simulink model "Simulation"  (R2025b)
settings: Solver=ode4  StartTime=0.0  StopTime=60  FixedStep=Ts  RelTol=1e-3
undefined symbols (not defined in the file or in its folder): A_SS_FD1, A_SS_FD3, A_zeta_f, A_zeta_tau, B_SS_FD1, B_SS_FD3, C_SS_FD1, C_SS_FD3, C_zeta_f, C_zeta_tau, D_SS_FD1, D_SS_FD3, eigs_NDO_force, eigs_NDO_torque, F1, F2, g_vec, inertia_factor, J, m, mass_factor, NDOB_force, NDOB_torque, period, radius, ReferenceTypeNumber, speed, Th_lower, Th_upper, Ts, Ts_hw, x0_FD1
libraries: simulink x9, dspstat3 x2
(part 1 of 2)
settings Model: SimulationMode=accelerator  SILPILSystemUnderTest=refmodels  Creator=baldo  LastModifiedBy=robyd
settings DebuggingCC: UnconnectedInputMsg=warning  UnconnectedOutputMsg=warning  UnconnectedLineMsg=warning
settings ModelReferenceCC: EnableRefExpFcnMdlSchedulingChecks=on
settings RTWCC: GPUComputeCapability=3.5  DLArmComputeVersion=19.05

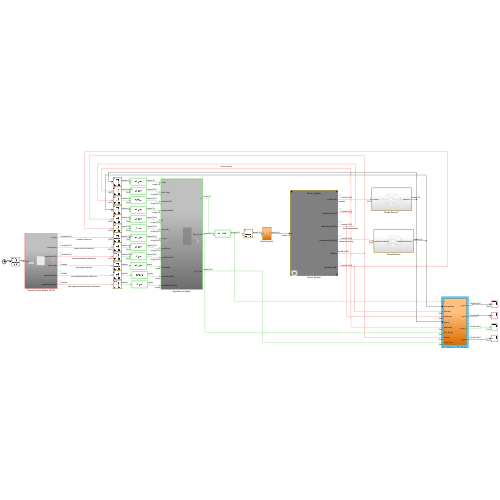
[thumbnail: Simulink's stored preview of the top-level diagram]
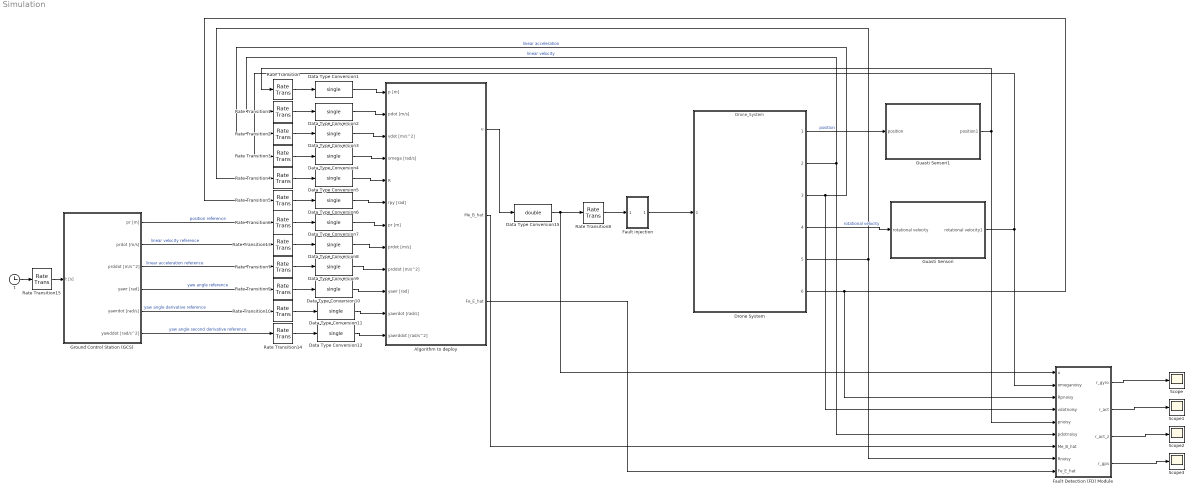
== system Simulation ==
  Algorithm to deploy : Subsystem
  Data Type Conversion{1..12} (12 alike) : DataTypeConversion  OutDataTypeStr=single  SaturateOnIntegerOverflow=off  RndMeth=Floor
  Data Type Conversion15 : DataTypeConversion  OutDataTypeStr=double  SaturateOnIntegerOverflow=off  RndMeth=Floor
  Drone System : ModelReference  ModelNameDialog=Drone_System  ModelReferenceVersion=9.10  CopyOfModelProtected=on
  Fault Detection (FD) Module : Subsystem
  Fault injection : Subsystem
  Ground Control Station (GCS) : Subsystem
  Guasti Sensori : Subsystem
  Guasti Sensori1 : Subsystem
  Rate Transition{,1..7,9..10,13..14} (12 alike) : RateTransition  OutPortSampleTime=Ts_hw
  Rate Transition15 : RateTransition  OutPortSampleTime=Ts
  Rate Transition8 : RateTransition  OutPortSampleTime=Ts
  Scope{,1..3} (4 alike) : Scope
      Scope settings: ActiveDisplayYMinimum=-1  ActiveDisplayYMaximum=1  DataLoggingVariableName=ScopeData5
      Scope1 settings: ActiveDisplayYMinimum=-1  ActiveDisplayYMaximum=1  DataLoggingVariableName=ScopeData7
      Scope2 settings: ActiveDisplayYMinimum=-1  ActiveDisplayYMaximum=1  DataLoggingVariableName=ScopeData8
      Scope3 settings: ActiveDisplayYMinimum=-1  ActiveDisplayYMaximum=1  DataLoggingVariableName=ScopeData9
  t : Clock
  wires:
  Algorithm to deploy/1(u) -> Data Type Conversion15/1
  Rate Transition/1 -> Data Type Conversion1/1
  Rate Transition1/1 -> Data Type Conversion2/1
  Rate Transition2/1 -> Data Type Conversion3/1
  Rate Transition3/1 -> Data Type Conversion4/1
  Rate Transition4/1 -> Data Type Conversion5/1
  Rate Transition5/1 -> Data Type Conversion6/1
  Rate Transition6/1 -> Data Type Conversion7/1
  Rate Transition13/1 -> Data Type Conversion8/1
  Rate Transition7/1 -> Data Type Conversion9/1
  Rate Transition9/1 -> Data Type Conversion10/1
  Rate Transition10/1 -> Data Type Conversion11/1
  Rate Transition14/1 -> Data Type Conversion12/1
  t/1 -> Rate Transition15/1
  Ground Control Station (GCS)/1(pr [m]) -> Rate Transition6/1  "position reference"
  Ground Control Station (GCS)/2(prdot [m/s]) -> Rate Transition13/1  "linear velocity reference"
  Ground Control Station (GCS)/3(prddot [m/s^2]) -> Rate Transition7/1  "linear acceleration reference"
  Ground Control Station (GCS)/4(yawr [rad]) -> Rate Transition9/1  "yaw angle reference"
  Ground Control Station (GCS)/5(yawrdot [rad/s]) -> Rate Transition10/1  "yaw angle derivative reference"
  Ground Control Station (GCS)/6(yawddot [rad/s^2]) -> Rate Transition14/1  "yaw angle second derivative reference"
  Data Type Conversion1/1 -> Algorithm to deploy/1(p [m])
  Data Type Conversion2/1 -> Algorithm to deploy/2(pdot [m/s])
  Data Type Conversion3/1 -> Algorithm to deploy/3(vdot [m/s^2])
  Data Type Conversion4/1 -> Algorithm to deploy/4(omega [rad/s])
  Data Type Conversion5/1 -> Algorithm to deploy/5(R)
  Data Type Conversion6/1 -> Algorithm to deploy/6(rpy [rad])
  Data Type Conversion7/1 -> Algorithm to deploy/7(pr [m])
  Data Type Conversion8/1 -> Algorithm to deploy/8(prdot [m/s])
  Data Type Conversion9/1 -> Algorithm to deploy/9(prddot [m/s^2])
  Data Type Conversion10/1 -> Algorithm to deploy/10(yawr [rad])
  Data Type Conversion11/1 -> Algorithm to deploy/11(yawrdot [rad/s])
  Data Type Conversion12/1 -> Algorithm to deploy/12(yawrddot [rad/s^2])
  Data Type Conversion15/1 -> Fault Detection (FD) Module/1(u), Rate Transition8/1
  Rate Transition15/1 -> Ground Control Station (GCS)/1(t [s])
  Drone System/2 -> Rate Transition1/1, Fault Detection (FD) Module/6(pdotnoisy)  "linear velocity"
  Drone System/3 -> Fault Detection (FD) Module/4(vdotnoisy), Rate Transition2/1  "linear acceleration"
  Drone System/5 -> Rate Transition4/1, Fault Detection (FD) Module/8(Rnoisy)
  Rate Transition8/1 -> Fault injection/1(In1)
  Fault injection/1(Out1) -> Drone System/1
  Drone System/4 -> Guasti Sensori/1(rotational velocity)  "rotational velocity"
  Guasti Sensori/1(rotational velocity1) -> Rate Transition3/1, Fault Detection (FD) Module/2(omeganoisy)
  Drone System/6 -> Fault Detection (FD) Module/3(Rpnoisy), Rate Transition5/1
  Drone System/1 -> Guasti Sensori1/1(position)  "position"
  Guasti Sensori1/1(position1) -> Fault Detection (FD) Module/5(pnoisy), Rate Transition/1
  Fault Detection (FD) Module/1(r_gyro) -> Scope/1
  Fault Detection (FD) Module/2(r_act) -> Scope1/1
  Fault Detection (FD) Module/3(r_act_z) -> Scope2/1
  Fault Detection (FD) Module/4(r_gps) -> Scope3/1
  Algorithm to deploy/2(Me_B_hat) -> Fault Detection (FD) Module/7(Me_B_hat)
  Algorithm to deploy/3(Fe_E_hat) -> Fault Detection (FD) Module/9(Fe_E_hat)

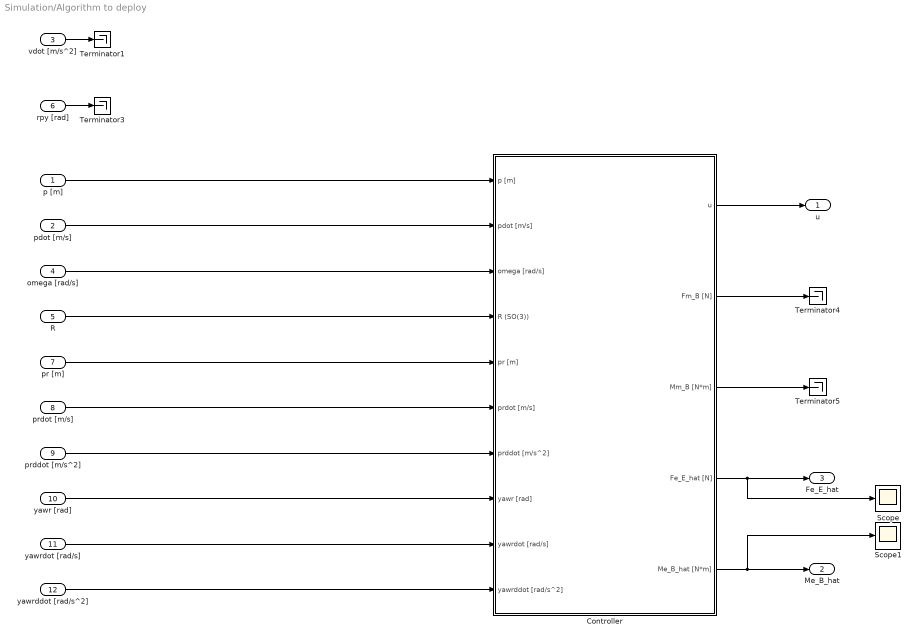
== system Simulation/Algorithm to deploy ==
  p [m] : Inport  OutDataTypeStr=single
  pdot [m/s] : Inport  Port=2  OutDataTypeStr=single
  vdot [m/s^2] : Inport  Port=3  OutDataTypeStr=single
  omega [rad/s] : Inport  Port=4  OutDataTypeStr=single
  R : Inport  Port=5  OutDataTypeStr=single
  rpy [rad] : Inport  Port=6  OutDataTypeStr=single
  pr [m] : Inport  Port=7  OutDataTypeStr=single
  prdot [m/s] : Inport  Port=8  OutDataTypeStr=single
  prddot [m/s^2] : Inport  Port=9  OutDataTypeStr=single
  yawr [rad] : Inport  Port=10  OutDataTypeStr=single
  yawrdot [rad/s] : Inport  Port=11  OutDataTypeStr=single
  yawrddot [rad/s^2] : Inport  Port=12  OutDataTypeStr=single
  Controller : Subsystem
  Scope : Scope
      settings: ActiveDisplayYMinimum=-18.049574136734009  ActiveDisplayYMaximum=25.171024560928345
  Scope1 : Scope
      settings: ActiveDisplayYMinimum=-0.31069509871304035  ActiveDisplayYMaximum=1.0718367416411638  DataLoggingVariableName=ScopeData2
  Terminator{1,3..5} (4 alike) : Terminator
  u : Outport  OutDataTypeStr=single
  Me_B_hat : Outport  Port=2  OutDataTypeStr=single
  Fe_E_hat : Outport  Port=3  OutDataTypeStr=single
  wires:
  vdot [m/s^2]/1 -> Terminator1/1
  rpy [rad]/1 -> Terminator3/1
  p [m]/1 -> Controller/1(p [m])
  pdot [m/s]/1 -> Controller/2(pdot [m/s])
  omega [rad/s]/1 -> Controller/3(omega [rad/s])
  R/1 -> Controller/4(R (SO(3)))
  pr [m]/1 -> Controller/5(pr [m])
  prdot [m/s]/1 -> Controller/6(prdot [m/s])
  prddot [m/s^2]/1 -> Controller/7(prddot [m/s^2])
  yawr [rad]/1 -> Controller/8(yawr [rad])
  yawrdot [rad/s]/1 -> Controller/9(yawrdot [rad/s])
  yawrddot [rad/s^2]/1 -> Controller/10(yawrddot [rad/s^2])
  Controller/1(u) -> u/1
  Controller/2(Fm_B [N]) -> Terminator4/1
  Controller/3(Mm_B [N*m]) -> Terminator5/1
  Controller/4(Fe_E_hat [N]) -> Fe_E_hat/1, Scope/1
  Controller/5(Me_B_hat [N*m]) -> Me_B_hat/1, Scope1/1

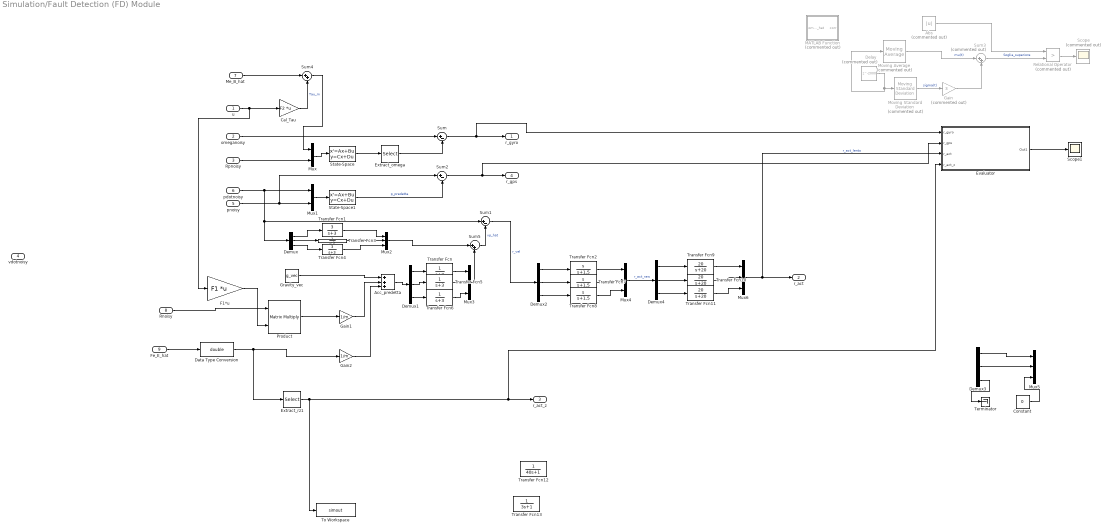
== system Simulation/Fault Detection (FD) Module ==
  u : Inport
  omeganoisy : Inport  Port=2
  Rpnoisy : Inport  Port=3
  vdotnoisy : Inport  Port=4
  pnoisy : Inport  Port=5
  pdotnoisy : Inport  Port=6
  Me_B_hat : Inport  Port=7
  Rnoisy : Inport  Port=8
  Fe_E_hat : Inport  Port=9
  Abs : Abs  Commented=on  SaturateOnIntegerOverflow=off
  Acc_predetta : Sum  Inputs=+++
  Cal_Tau : Gain  Gain=F2  Multiplication=Matrix(K*u)
  Constant : Constant  Value=0
  Data Type Conversion : DataTypeConversion  OutDataTypeStr=double  SaturateOnIntegerOverflow=off  RndMeth=Floor
  Delay : Delay  Commented=on  DelayLength=2000
  Demux{,1..4} (5 alike) : Demux  Outputs=3
  Evaluator : Subsystem
  Extract_omega : Selector  InputPortWidth=6  IndexOptions=Index vector (dialog)  Indices=[4 5 6]  OutputSizes=1
  Extract_rz1 : Selector  InputPortWidth=3  IndexOptions=Index vector (dialog)  Indices=[3]  OutputSizes=1
  F1*u : Gain  Gain=F1  Multiplication=Matrix(K*u)
  Gain : Gain  Commented=on  Gain=3
  Gain1 : Gain  Gain=1/m
  Gain2 : Gain  Gain=1/m
  Gravity_vec : Constant  Value=g_vec
  MATLAB Function : MATLAB Function  Commented=on  TreatAsAtomicUnit=on
  Moving Average : dspstat3/Moving Average  Commented=on  Method=Sliding window  ForgettingFactorPort=off  SpecifyWindowLength=on  WindowLength=2000  OverlapLength=3  AllowArbitraryInputLength=off  ForgettingFactor=0.9  SimulateUsing=Interpreted execution
  Moving Standard Deviation : dspstat3/Moving Standard Deviation  Commented=on  Method=Sliding window  ForgettingFactorPort=off  SpecifyWindowLength=on  WindowLength=2000  OverlapLength=3  AllowArbitraryInputLength=off  ForgettingFactor=0.9  SimulateUsing=Interpreted execution
  Mux : Mux  Inputs=2
  Mux1 : Mux  Inputs=2
  Mux{2..6} (5 alike) : Mux  Inputs=3
  Product : Product  Multiplication=Matrix(*)
  Relational Operator : RelationalOperator  Commented=on  Operator=>  OutDataTypeStr=boolean  RndMeth=Simplest  InputSameDT=off
  Scope : Scope  Commented=on
      settings: DataLoggingVariableName=ScopeData10
  Scope1 : Scope
      settings: ActiveDisplayYMinimum=-1  ActiveDisplayYMaximum=1  DataLoggingVariableName=ScopeData11
  State-Space : StateSpace  A=A_SS_FD1  B=B_SS_FD1  C=C_SS_FD1  D=D_SS_FD1  InitialCondition=x0_FD1
  State-Space1 : StateSpace  A=A_SS_FD3  B=B_SS_FD3  C=C_SS_FD3  D=D_SS_FD3  InitialCondition=0
  Sum : Sum  Inputs=|+-
  Sum1 : Sum  Inputs=|+-
  Sum2 : Sum  Inputs=|+-
  Sum3 : Sum  Commented=on  Inputs=|++
  Sum4 : Sum  Inputs=|++
  Sum5 : Sum  Inputs=|++
  Terminator : Terminator
  To Workspace : ToWorkspace  VariableName=simout  SaveFormat=Timeseries  SampleTime=-1
  Transfer Fcn : TransferFcn  Denominator=[1 3]
  Transfer Fcn1 : TransferFcn  Numerator=[3]  Denominator=[1 3]
  Transfer Fcn10 : TransferFcn  Numerator=[20]  Denominator=[1 20]
  Transfer Fcn11 : TransferFcn  Numerator=[20]  Denominator=[1 20]
  Transfer Fcn12 : TransferFcn  Denominator=[40 1]
  Transfer Fcn13 : TransferFcn  Denominator=[3 1]
  Transfer Fcn2 : TransferFcn  Numerator=[1 0]  Denominator=[1 1.5]
  Transfer Fcn3 : TransferFcn  Numerator=[3]  Denominator=[1 3]
  Transfer Fcn4 : TransferFcn  Numerator=[3]  Denominator=[1 3]
  Transfer Fcn5 : TransferFcn  Denominator=[1 3]
  Transfer Fcn6 : TransferFcn  Denominator=[1 3]
  Transfer Fcn7 : TransferFcn  Numerator=[1 0]  Denominator=[1 1.5]
  Transfer Fcn8 : TransferFcn  Numerator=[1 0]  Denominator=[1 1.5]
  Transfer Fcn9 : TransferFcn  Numerator=[20]  Denominator=[1 20]
  r_gyro : Outport
  r_act : Outport  Port=2
  r_act_z : Outport  Port=3
  r_gps : Outport  Port=4
  wires:
  u/1 -> Cal_Tau/1, F1*u/1
  Cal_Tau/1 -> Sum4/2  "Tau_m"
  Rpnoisy/1 -> Mux/2
  Mux/1 -> State-Space/1
  State-Space/1 -> Extract_omega/1
  omeganoisy/1 -> Sum/1
  Extract_omega/1 -> Sum/2
  Sum/1 -> Evaluator/1(r_gyro), r_gyro/1
  Gravity_vec/1 -> Acc_predetta/1
  F1*u/1 -> Product/2
  Sum1/1 -> Demux2/1  "r_vel"
  pnoisy/1 -> Mux1/2, Sum2/1
  pdotnoisy/1 -> Demux/1, Sum1/1, Mux1/1
  Mux1/1 -> State-Space1/1
  State-Space1/1 -> Sum2/2  "p_predetta"
  Sum2/1 -> Evaluator/2(r_gps), r_gps/1
  Moving Average/1 -> Sum3/1  "mu(t)"
  Moving Standard Deviation/1 -> Gain/1  "sigma(t)"
  Gain/1 -> Sum3/2
  Sum3/1 -> Relational Operator/2  "Soglia_superiore"
  Abs/1 -> Relational Operator/1
  Delay/1 -> Moving Standard Deviation/1, Moving Average/1
  Relational Operator/1 -> Scope/1
  Evaluator/1(Out1) -> Scope1/1
  Me_B_hat/1 -> Sum4/1
  Sum4/1 -> Mux/1
  Rnoisy/1 -> Product/1
  Product/1 -> Gain1/1
  Fe_E_hat/1 -> Data Type Conversion/1
  Gain1/1 -> Acc_predetta/2
  Gain2/1 -> Acc_predetta/3
  Sum5/1 -> Sum1/2  "vp_hat"
  Transfer Fcn1/1 -> Mux2/1
  Demux/1 -> Transfer Fcn1/1
  Demux/2 -> Transfer Fcn3/1
  Transfer Fcn3/1 -> Mux2/2
  Demux/3 -> Transfer Fcn4/1
  Transfer Fcn4/1 -> Mux2/3
  Mux2/1 -> Sum5/1
  Acc_predetta/1 -> Demux1/1
  Transfer Fcn/1 -> Mux3/1
  Demux1/1 -> Transfer Fcn/1
  Demux1/2 -> Transfer Fcn5/1
  Transfer Fcn5/1 -> Mux3/2
  Demux1/3 -> Transfer Fcn6/1
  Transfer Fcn6/1 -> Mux3/3
  Mux3/1 -> Sum5/2
  Demux2/1 -> Transfer Fcn2/1
  Transfer Fcn2/1 -> Mux4/1
  Demux2/2 -> Transfer Fcn7/1
  Transfer Fcn7/1 -> Mux4/2
  Demux2/3 -> Transfer Fcn8/1
  Transfer Fcn8/1 -> Mux4/3
  Data Type Conversion/1 -> Extract_rz1/1, Gain2/1
  Demux3/1 -> Mux5/1
  Demux3/2 -> Mux5/2
  Demux3/3 -> Terminator/1
  Constant/1 -> Mux5/3
  Demux4/2 -> Transfer Fcn10/1
  Transfer Fcn10/1 -> Mux6/2
  Demux4/1 -> Transfer Fcn9/1
  Transfer Fcn9/1 -> Mux6/1
  Demux4/3 -> Transfer Fcn11/1
  Mux4/1 -> Demux4/1  "r_act_raw"
  Transfer Fcn11/1 -> Mux6/3
  Mux6/1 -> r_act/1, Evaluator/3(r_act)  "r_act_lento"
  Extract_rz1/1 -> Evaluator/4(r_act_z), r_act_z/1, To Workspace/1

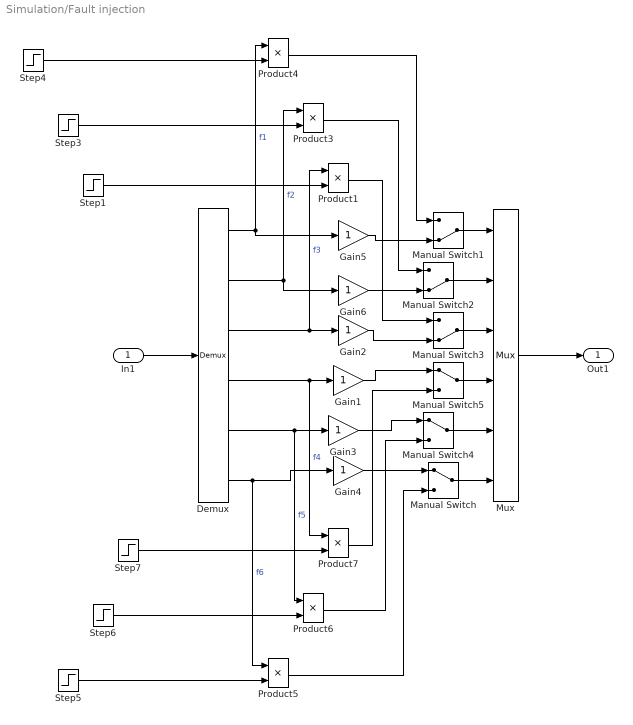
== system Simulation/Fault injection ==
  In1 : Inport
  Demux : Demux  Outputs=6
  Gain{1..6} (6 alike) : Gain
  Manual Switch : ManualSwitch
  Manual Switch1 : ManualSwitch  CurrentSetting=0
  Manual Switch2 : ManualSwitch  CurrentSetting=0
  Manual Switch3 : ManualSwitch  CurrentSetting=0
  Manual Switch4 : ManualSwitch
  Manual Switch5 : ManualSwitch
  Mux : Mux  Inputs=6
  Product{1,3..7} (6 alike) : Product
  Step{1,3,5..7} (5 alike) : Step  Time=20  Before=1  After=0.4  SampleTime=0
  Step4 : Step  Time=20  Before=1  After=0.8  SampleTime=0
  Out1 : Outport
  wires:
  Demux/3 -> Product1/1, Gain2/1  "f3"
  In1/1 -> Demux/1
  Mux/1 -> Out1/1
  Demux/4 -> Gain1/1, Product7/1  "f4"
  Demux/5 -> Product6/1, Gain3/1  "f5"
  Step1/1 -> Product1/2
  Demux/6 -> Product5/1, Gain4/1  "f6"
  Manual Switch/1 -> Mux/6
  Gain4/1 -> Manual Switch/1
  Manual Switch1/1 -> Mux/1
  Gain5/1 -> Manual Switch1/2
  Manual Switch2/1 -> Mux/2
  Gain6/1 -> Manual Switch2/2
  Manual Switch3/1 -> Mux/3
  Manual Switch4/1 -> Mux/5
  Manual Switch5/1 -> Mux/4
  Gain2/1 -> Manual Switch3/2
  Gain1/1 -> Manual Switch5/1
  Gain3/1 -> Manual Switch4/1
  Demux/1 -> Product4/1, Gain5/1  "f1"
  Demux/2 -> Gain6/1, Product3/1  "f2"
  Step3/1 -> Product3/2
  Step4/1 -> Product4/2
  Step6/1 -> Product6/2
  Step7/1 -> Product7/2
  Step5/1 -> Product5/2
  Product7/1 -> Manual Switch5/2
  Product6/1 -> Manual Switch4/2
  Product5/1 -> Manual Switch/2
  Product1/1 -> Manual Switch3/1
  Product3/1 -> Manual Switch2/1
  Product4/1 -> Manual Switch1/1

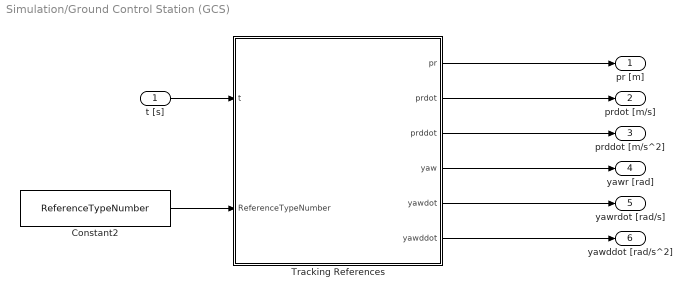
== system Simulation/Ground Control Station (GCS) ==
  t [s] : Inport
  Constant2 : Constant  Value=ReferenceTypeNumber  SampleTime=Ts
  Tracking References : MATLAB Function  TreatAsAtomicUnit=on
  pr [m] : Outport
  prdot [m/s] : Outport  Port=2
  prddot [m/s^2] : Outport  Port=3
  yawr [rad] : Outport  Port=4
  yawrdot [rad/s] : Outport  Port=5
  yawddot [rad/s^2] : Outport  Port=6
  wires:
  Tracking References/5(yawdot) -> yawrdot [rad/s]/1
  Tracking References/6(yawddot) -> yawddot [rad/s^2]/1
  Tracking References/3(prddot) -> prddot [m/s^2]/1
  Tracking References/2(prdot) -> prdot [m/s]/1
  Tracking References/4(yaw) -> yawr [rad]/1
  Tracking References/1(pr) -> pr [m]/1
  t [s]/1 -> Tracking References/1(t)
  Constant2/1 -> Tracking References/2(ReferenceTypeNumber)

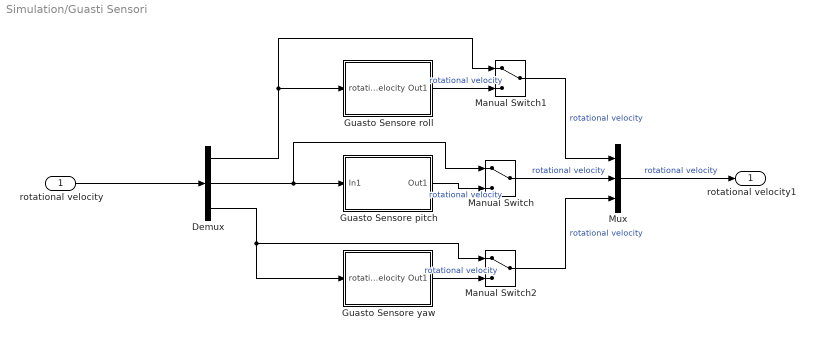
== system Simulation/Guasti Sensori ==
  rotational velocity : Inport
  Demux : Demux  Outputs=3
  Guasto Sensore pitch : Subsystem
  Guasto Sensore roll : Subsystem
  Guasto Sensore yaw : Subsystem
  Manual Switch : ManualSwitch
  Manual Switch1 : ManualSwitch
  Manual Switch2 : ManualSwitch
  Mux : Mux  Inputs=3
  rotational velocity1 : Outport
  wires:
  Manual Switch1/1 -> Mux/1  "rotational velocity"
  Guasto Sensore pitch/1(Out1) -> Manual Switch/2  "rotational velocity"
  Manual Switch/1 -> Mux/2  "rotational velocity"
  Manual Switch2/1 -> Mux/3  "rotational velocity"
  Mux/1 -> rotational velocity1/1  "rotational velocity"
  Guasto Sensore yaw/1(Out1) -> Manual Switch2/2  "rotational velocity"
  Guasto Sensore roll/1(Out1) -> Manual Switch1/2  "rotational velocity"
  rotational velocity/1 -> Demux/1
  Demux/2 -> Manual Switch/1, Guasto Sensore pitch/1(In1)
  Demux/1 -> Manual Switch1/1, Guasto Sensore roll/1(rotational velocity)
  Demux/3 -> Manual Switch2/1, Guasto Sensore yaw/1(rotational velocity)

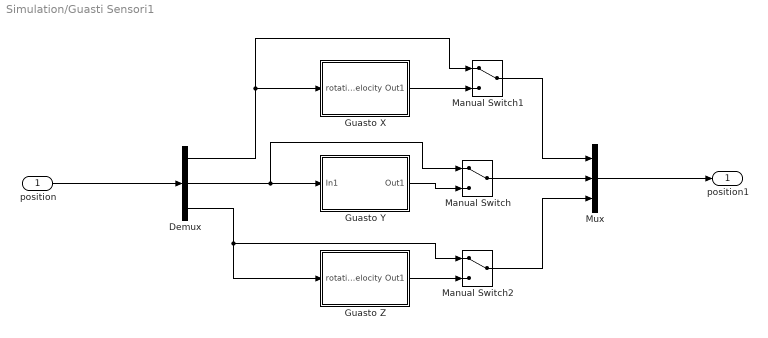
== system Simulation/Guasti Sensori1 ==
  position : Inport
  Demux : Demux  Outputs=3
  Guasto X : Subsystem
  Guasto Y : Subsystem
  Guasto Z : Subsystem
  Manual Switch : ManualSwitch
  Manual Switch1 : ManualSwitch
  Manual Switch2 : ManualSwitch
  Mux : Mux  Inputs=3
  position1 : Outport
  wires:
  Manual Switch1/1 -> Mux/1
  Guasto Y/1(Out1) -> Manual Switch/2
  Manual Switch/1 -> Mux/2
  Manual Switch2/1 -> Mux/3
  Mux/1 -> position1/1
  Guasto Z/1(Out1) -> Manual Switch2/2
  Guasto X/1(Out1) -> Manual Switch1/2
  position/1 -> Demux/1
  Demux/2 -> Manual Switch/1, Guasto Y/1(In1)
  Demux/1 -> Manual Switch1/1, Guasto X/1(rotational velocity)
  Demux/3 -> Manual Switch2/1, Guasto Z/1(rotational velocity)

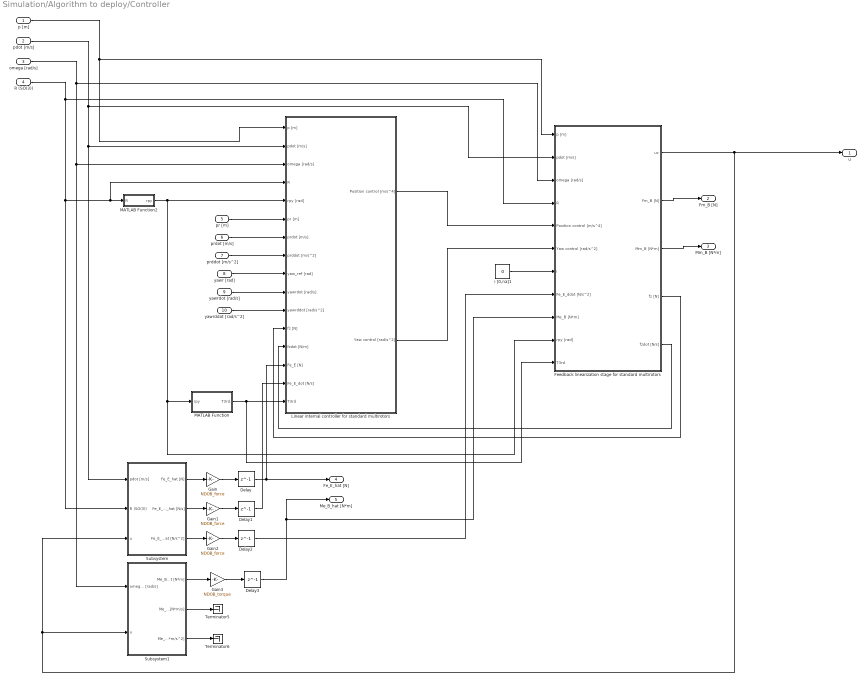
== system Simulation/Algorithm to deploy/Controller ==
  p [m] : Inport
  pdot [m/s] : Inport  Port=2
  omega [rad/s] : Inport  Port=3
  R (SO(3)) : Inport  Port=4
  pr [m] : Inport  Port=5  OutDataTypeStr=single
  prdot [m/s] : Inport  Port=6  OutDataTypeStr=single
  prddot [m/s^2] : Inport  Port=7  OutDataTypeStr=single
  yawr [rad] : Inport  Port=8  OutDataTypeStr=single
  yawrdot [rad/s] : Inport  Port=9  OutDataTypeStr=single
  yawrddot [rad/s^2] : Inport  Port=10  OutDataTypeStr=single
  Delay{,1..3} (4 alike) : Delay  DelayLength=1  InitialCondition=0
  Feedback linearization stage for standard multirotors : Subsystem  mask{mask_m=single(m*mass_factor), mask_J=single(J*inertia_factor), mask_rg_B=zeros(3,1), mask_F1=single(F1), mask_F2=single(F2), mask_thrustmax=1, mask_fz0=single(m*9.8), mask_Ts=Ts_hw}
      mask prompts: mask_m "Mass [kg]"; mask_J "Inertia Tensor [kg*m^2]"; mask_rg_B "Center of mass [m]"; mask_F1 "Control force input matrix"; mask_F2 "Control moment input matrix"; mask_thrustmax "Max thrust [N]"; mask_fz0 "Upward lift force"; mask_Ts "Sample time"
      mask init:
      | % Wrappers
      |     e1 = single([1; 0; 0]);
      |     e2 = single([0; 1; 0]);
      |     e3 = single([0; 0; 1]);
      |     
      |     %%%%%%%%%%%%%%%%%%%%%%%%%%%%%%%%%%%%%%%%%%%%
      |     %    Some general paramater
      |     %%%%%%%%%%%%%%%%%%%%%%%%%%%%%%%%%%%%%%%%%%%%
      |     mask_Jinv = inv(mask_J);
      |     mask_g = single(9.8);
      |     mask_na = size(mask_F1,2);
      | 
      |     %%%%%%%%%%%%%%%%%%%%%%%%%%%%%%%%%%%%%%%%%%%%
      |     %    Allocation for standard multirotors
      |     %%%%%%%%%%%%%%%%%%%%%%%%%%%%%%%%%%%%%%%%%%%%
      |     A = [mask_F1(3,:); mask_F2];
      |     A_pinv = single(pinv(A));
      mask DialogControl DescGroupVar Prompt: Feedback linearization stage for standard multirotors
      mask DialogControl DescTextVar Prompt: Dynamic feedback linearization for standard multirotors. Moore-Penrose allocation. The dynamic estension is "exact".
      mask DialogControl Control3 Prompt: Author: Alessandro Baldini
      mask DialogControl ParameterGroupVar Prompt: Multirotor parameters
      mask DialogControl Container4 Prompt: Initial condition and others
  Gain : Gain  Gain=NDOB_force
  Gain1 : Gain  Gain=NDOB_force
  Gain2 : Gain  Gain=NDOB_force
  Gain3 : Gain  Gain=NDOB_torque
  Linear internal controller for standard multirotors : Subsystem  mask{mask_m=single(m*mass_factor), mask_J=single(J*inertia_factor), mask_rg_B=zeros(3,1), mask_F1=single(F1), mask_F2=single(F2), mask_thrustmax=1, mask_xpoles=single([-3.0 -3.1 -3.2 -3.2 -1.3]/1.3), mask_ypoles=single([-3.0 -3.1 -3.2 -3.2 -1.3]/1.3), mask_zpoles=single([-3.0 -3.1 -3.2 -3.2 -1.3]/1.3), mask_yawpoles=single([-1 -2]), mask_chkPID=off, mask_chkYaw=off, mask_fz0=single(m*9.8), mask_Ts=Ts_hw}
      mask prompts: mask_m "Mass [kg]"; mask_J "Inertia Tensor [kg*m^2]"; mask_rg_B "Center of mass [m]"; mask_F1 "Control force input matrix"; mask_F2 "Control moment input matrix"; mask_thrustmax "Max thrust [N]"; mask_xpoles "Closed loop x poles"; mask_ypoles "Closed loop y poles"; mask_zpoles "Closed loop z poles"; mask_yawpoles "Closed loop yaw poles"; mask_chkPID "Enable position integrators"; mask_chkYaw "Enable yaw integrator"; mask_fz0 "Upward lift force"; mask_Ts "Sample time"
      mask init:
      | % Wrappers
      |     e1 = [1; 0; 0];
      |     e2 = [0; 1; 0];
      |     e3 = [0; 0; 1];
      |     
      |     %%%%%%%%%%%%%%%%%%%%%%%%%%%%%%%%%%%%%%%%%%%%
      |     %    Some general paramater
      |     %%%%%%%%%%%%%%%%%%%%%%%%%%%%%%%%%%%%%%%%%%%%
      |     mask_Jinv = inv(mask_J);
      |     mask_g = 9.8;
      |     mask_na = size(mask_F1,2);
      |     
      |     %%%%%%%%%%%%%%%%%%%%%%%%%%%%%%%%%%%%%%%%%%%%
      |     %    ( Control paramaters)
      |     %%%%%%%%%%%%%%%%%%%%%%%%%%%%%%%%%%%%%%%%%%%%
      |     % Calculation of outer loop parameters
      |     polyx = poly(mask_xpoles);
      |     polyy = poly(mask_ypoles);
      |     polyz = poly(mask_zpoles);
      |     polyyaw = poly(mask_yawpoles);
      | 
      |     if mask_chkPID == 1
      |         % Raw pole placement (with integral action)
      |         % We consider the first 5 poles (2 for yaw)
      |         mask_xpoles = mask_xpoles(1:5);
      |         mask_ypoles = mask_ypoles(1:5);
      |         mask_zpoles = mask_zpoles(1:5);
      |         polyyaw = polyyaw(1:2);
      | 
      |         polyx = poly(mask_xpoles);
      |         polyy = poly(mask_ypoles);
      |         polyz = poly(mask_zpoles);
      |         polyyaw = poly(mask_yawpoles);
      | 
      |         mask_k0 = diag([polyx(6) polyy(6) polyz(6)]);
      |         mask_k1 = diag([polyx(5) polyy(5) polyz(5)]);
      |         mask_k2 = diag([polyx(4) polyy(4) polyz(4)]);
      |         mask_k3 = diag([polyx(3) polyy(3) polyz(3)]);
      |         mask_k4 = diag([polyx(2) polyy(2) polyz(2)]);
      |         
      |         k0yaw = polyyaw(3);
      |         k1yaw = polyyaw(2);
      | 
      |     else
      |         % Raw pole placement (no integral action)
      |         % We consider the first 4 poles (2 for yaw)
      |         mask_xpoles = mask_xpoles(1:4);
      |         mask_ypoles = mask_ypoles(1:4);
      |         mask_zpoles = mask_zpoles(1:4);
      |         polyyaw = polyyaw(1:2);
      | 
      |         polyx = poly(mask_xpoles);
      |         polyy = poly(mask_ypoles);
      |         polyz = poly(mask_zpoles);
      |         polyyaw = poly(mask_yawpoles);
      | 
      |         mask_k0 = diag([polyx(5) polyy(5) polyz(5)]);
      |         mask_k1 = diag([polyx(4) polyy(4) polyz(4)]);
      |         mask_k2 = diag([polyx(3) polyy(3) polyz(3)]);
      |         mask_k3 = diag([polyx(2) polyy(2) polyz(2)]);
      |         mask_k4 = zeros(1,3); % Not used in this control mode
      | 
      |         k0yaw = polyyaw(3);
      |         k1yaw = polyyaw(2);
      |     end
      mask DialogControl DescGroupVar Prompt: Linear controller for standard multirotors
      mask DialogControl DescTextVar Prompt: Linear state space pole placement to couple with a feedback linearization stage. For standard multirotors.
      mask DialogControl Control3 Prompt: Author: Alessandro Baldini
      mask DialogControl ParameterGroupVar Prompt: Multirotor parameters
      mask DialogControl Container3 Prompt: Control paramaters (+1 pole each in case of integrators)
      mask DialogControl Container4 Prompt: Initial condition and others
  MATLAB Function : MATLAB Function  TreatAsAtomicUnit=on
  MATLAB Function2 : MATLAB Function  TreatAsAtomicUnit=on
  Subsystem : Subsystem  mask{mask_m=single(m*mass_factor), mask_F1=single(F1), mask_C=single(C_zeta_f), mask_A=single(A_zeta_f), mask_poles=single(eigs_NDO_force), mask_Ts=Ts_hw}
      mask prompts: mask_m "Mass [kg]"; mask_F1 "Control force input matrix"; mask_C "Exogenous system output matrix C"; mask_A "Exogenous system dynamics matrix A"; mask_poles "Poles to place"; mask_Ts "Sample time"
      mask init:
      | mask_nzeta = size(mask_A,2);
      |     if length(mask_poles) < mask_nzeta
      |         error(num2str(mask_nzeta) + " poles should be specified for the force estimation.")
      |     end
      | 
      |     mask_H = place(mask_A',mask_C',mask_poles(1:mask_nzeta))';
      |     mask_AH = mask_A - mask_H*mask_C;
      |     mask_g = 9.8;
      mask DialogControl DescGroupVar Prompt: Rigid body force observer - v 0.1
      mask DialogControl DescTextVar Prompt: Force observer for a rigid body through a Nonlinear Disturbance Observer (NDO), i.e., reduced order functional observer.
      mask DialogControl Control2 Prompt: Author: Alessandro Baldini
      mask DialogControl Mask_marameters Prompt: Parameters
      mask DialogControl Container3 Prompt: Initial conditions and others
  Subsystem1 : Subsystem  mask{mask_J=single(J*inertia_factor), mask_F2=single(F2), mask_C=single(C_zeta_tau), mask_A=single(A_zeta_tau), mask_poles=single(eigs_NDO_torque), mask_Ts=Ts_hw}
      mask prompts: mask_J "Inertia tensor [kg*m^2]"; mask_F2 "Control moment input matrix"; mask_C "Exogenous system output matrix C"; mask_A "Exogenous system dynamics matrix A"; mask_poles "Poles to place"; mask_Ts "Sample time"
      mask init:
      | mask_nzeta = size(mask_A,2);
      |     if length(mask_poles) < mask_nzeta
      |         error(num2str(mask_nzeta) + " poles should be specified for the torque estimation.")
      |     end
      | 
      |     mask_H = place(mask_A',mask_C',mask_poles(1:mask_nzeta))';
      |     mask_AH = mask_A - mask_H*mask_C;
      mask DialogControl DescGroupVar Prompt: Rigid body torque observer - v 0.1
      mask DialogControl DescTextVar Prompt: Torque observer for a rigid body through a Nonlinear Disturbance Observer (NDO), i.e., reduced order functional observer.
      mask DialogControl Control2 Prompt: Author: Alessandro Baldini
      mask DialogControl Mask_marameters Prompt: Parameters
      mask DialogControl Container3 Prompt: Initial conditions and others
  Terminator5 : Terminator
  Terminator6 : Terminator
  i [0,na]1 : Constant  Value=0  OutDataTypeStr=single  SampleTime=Ts_hw
  u : Outport
  Fm_B [N] : Outport  Port=2
  Mm_B [N*m] : Outport  Port=3
  Fe_E_hat [N] : Outport  Port=4  OutDataTypeStr=single
  Me_B_hat [N*m] : Outport  Port=5  OutDataTypeStr=single
  wires:
  Feedback linearization stage for standard multirotors/2(Fm_B [N]) -> Fm_B [N]/1
  pr [m]/1 -> Linear internal controller for standard multirotors/6(pr [m])
  Linear internal controller for standard multirotors/2(" Yaw control [rad/s^2]") -> Feedback linearization stage for standard multirotors/6(Yaw control [rad/s^2])
  pdot [m/s]/1 -> Feedback linearization stage for standard multirotors/2(pdot [m/s]), Subsystem/1(pdot [m/s]), Linear internal controller for standard multirotors/2(pdot [m/s])
  Delay2/1 -> Feedback linearization stage for standard multirotors/8(Fe_E_ddot [N/s^2])
  Delay/1 -> Fe_E_hat [N]/1, Linear internal controller for standard multirotors/14(Fe_E [N])
  MATLAB Function/1(T3rd) -> Feedback linearization stage for standard multirotors/11(T3rd), Linear internal controller for standard multirotors/16(T3rd)
  Delay1/1 -> Linear internal controller for standard multirotors/15(Fe_E_dot [N/s])
  yawr [rad]/1 -> Linear internal controller for standard multirotors/9(yaw_ref [rad])
  MATLAB Function2/1(rpy) -> Linear internal controller for standard multirotors/5(rpy [rad]), Feedback linearization stage for standard multirotors/10(rpy [rad]), MATLAB Function/1(rpy)
  Gain/1 -> Delay/1
  prdot [m/s]/1 -> Linear internal controller for standard multirotors/7(prdot [m/s])
  Feedback linearization stage for standard multirotors/5(fzdot [N/s]) -> Linear internal controller for standard multirotors/13(fzdot [N/m])
  Feedback linearization stage for standard multirotors/4(fz [N]) -> Linear internal controller for standard multirotors/12(fz [N])
  R (SO(3))/1 -> Feedback linearization stage for standard multirotors/4(R), Linear internal controller for standard multirotors/4(R), MATLAB Function2/1(R), Subsystem/2(R (SO(3)))
  Subsystem1/3(Me_B_ddot_hat [N*m/s^2]) -> Terminator6/1
  Subsystem/3(Fe_E_ddot_hat [N/s^2]) -> Gain2/1
  Feedback linearization stage for standard multirotors/1(uc) -> u/1, Subsystem/3(u), Subsystem1/2(u)
  Subsystem/2(Fe_E_dot_hat [N/s]) -> Gain1/1
  Subsystem/1(Fe_E_hat [N]) -> Gain/1
  Gain1/1 -> Delay1/1
  Linear internal controller for standard multirotors/1(" Position control [m/s^4]") -> Feedback linearization stage for standard multirotors/5(Position control [m/s^4])
  Subsystem1/1(Me_B_hat [N*m]) -> Gain3/1
  omega [rad/s]/1 -> Subsystem1/1(omega [rad/s]), Linear internal controller for standard multirotors/3(omega [rad/s]), Feedback linearization stage for standard multirotors/3(omega [rad/s])
  yawrdot [rad/s]/1 -> Linear internal controller for standard multirotors/10(yawrdot [rad/s])
  yawrddot [rad/s^2]/1 -> Linear internal controller for standard multirotors/11(yawrddot [rad/s^2])
  p [m]/1 -> Linear internal controller for standard multirotors/1(p [m]), Feedback linearization stage for standard multirotors/1(p [m])
  prddot [m/s^2]/1 -> Linear internal controller for standard multirotors/8(prddot [m/s^2])
  Feedback linearization stage for standard multirotors/3(Mm_B [N*m]) -> Mm_B [N*m]/1
  Subsystem1/2(Me_B_dot_hat [N*m/s]) -> Terminator5/1
  Gain2/1 -> Delay2/1
  Delay3/1 -> Me_B_hat [N*m]/1, Feedback linearization stage for standard multirotors/9(Me_B [N*m])
  Gain3/1 -> Delay3/1
  i [0,na]1/1 -> Feedback linearization stage for standard multirotors/7(i)

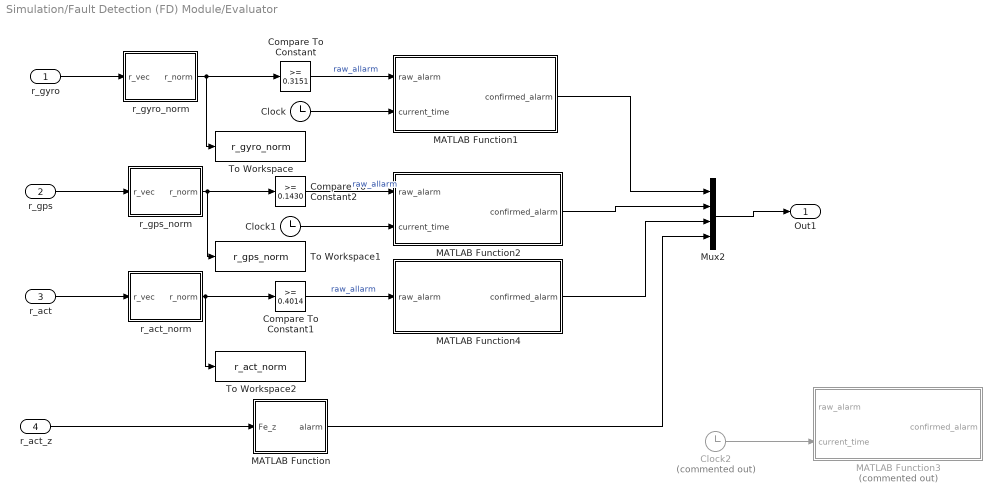
== system Simulation/Fault Detection (FD) Module/Evaluator ==
  r_gyro : Inport
  r_gps : Inport  Port=2
  r_act : Inport  Port=3
  r_act_z : Inport  Port=4
  Clock : Clock
  Clock1 : Clock
  Clock2 : Clock  Commented=on
  Compare To Constant : simulink/Logic and Bit Operations/Compare To Constant  relop=>=  const=0.3151  OutDataTypeStr=boolean
  Compare To Constant1 : simulink/Logic and Bit Operations/Compare To Constant  relop=>=  const=0.4014  OutDataTypeStr=boolean
  Compare To Constant2 : simulink/Logic and Bit Operations/Compare To Constant  relop=>=  const=0.1430  OutDataTypeStr=boolean
  MATLAB Function : MATLAB Function  TreatAsAtomicUnit=on
  MATLAB Function1 : MATLAB Function  TreatAsAtomicUnit=on
  MATLAB Function2 : MATLAB Function  TreatAsAtomicUnit=on
  MATLAB Function3 : MATLAB Function  Commented=on  TreatAsAtomicUnit=on
  MATLAB Function4 : MATLAB Function  TreatAsAtomicUnit=on
  Mux2 : Mux
  To Workspace : ToWorkspace  VariableName=r_gyro_norm  SaveFormat=Timeseries  SampleTime=-1
  To Workspace1 : ToWorkspace  VariableName=r_gps_norm  SaveFormat=Timeseries  SampleTime=-1
  To Workspace2 : ToWorkspace  VariableName=r_act_norm  SaveFormat=Timeseries  SampleTime=-1
  r_act_norm : MATLAB Function  TreatAsAtomicUnit=on
  r_gps_norm : MATLAB Function  TreatAsAtomicUnit=on
  r_gyro_norm : MATLAB Function  TreatAsAtomicUnit=on
  Out1 : Outport
  wires:
  Clock/1 -> MATLAB Function1/2(current_time)
  Compare To Constant1/1 -> MATLAB Function4/1(raw_alarm)  "raw_allarm"
  r_gps/1 -> r_gps_norm/1(r_vec)
  r_gps_norm/1(r_norm) -> To Workspace1/1, Compare To Constant2/1
  MATLAB Function2/1(confirmed_alarm) -> Mux2/2
  Clock2/1 -> MATLAB Function3/2(current_time)
  MATLAB Function1/1(confirmed_alarm) -> Mux2/1
  r_gyro_norm/1(r_norm) -> To Workspace/1, Compare To Constant/1
  r_act_norm/1(r_norm) -> To Workspace2/1, Compare To Constant1/1
  Compare To Constant/1 -> MATLAB Function1/1(raw_alarm)  "raw_allarm"
  r_act/1 -> r_act_norm/1(r_vec)
  Clock1/1 -> MATLAB Function2/2(current_time)
  Compare To Constant2/1 -> MATLAB Function2/1(raw_alarm)  "raw_allarm"
  r_gyro/1 -> r_gyro_norm/1(r_vec)
  Mux2/1 -> Out1/1
  MATLAB Function4/1(confirmed_alarm) -> Mux2/3
  r_act_z/1 -> MATLAB Function/1(Fe_z)
  MATLAB Function/1(alarm) -> Mux2/4

== system Simulation/Guasti Sensori/Guasto Sensore pitch ==
  In1 : Inport
  Add : Sum
  Ramp : simulink/Sources/Ramp  slope=0.01  start=20  InitialOutput=0
  Saturation : Saturate  UpperLimit=5  LowerLimit=-5
  Scope : Scope
      settings: ActiveDisplayYMinimum=-1  ActiveDisplayYMaximum=1  DataLoggingVariableName=ScopeData3
  Scope1 : Scope
      settings: ActiveDisplayYMinimum=-0.55531902367440134  ActiveDisplayYMaximum=0.70340368575655188  DataLoggingVariableName=ScopeData4
  Out1 : Outport
  wires:
  Add/1 -> Scope/1, Out1/1
  In1/1 -> Scope1/1, Add/1
  Ramp/1 -> Saturation/1
  Saturation/1 -> Add/2

== system Simulation/Guasti Sensori/Guasto Sensore roll ==
  rotational velocity : Inport
  Add : Sum
  Ramp : simulink/Sources/Ramp  slope=0.01  start=20  InitialOutput=0
  Saturation : Saturate  UpperLimit=5  LowerLimit=-5
  Scope : Scope
      settings: ActiveDisplayYMinimum=-0.47156763154329079  ActiveDisplayYMaximum=0.958434860305525  DataLoggingVariableName=ScopeData3
  Scope1 : Scope
      settings: ActiveDisplayYMinimum=-0.55531902367440134  ActiveDisplayYMaximum=0.70340368575655188  DataLoggingVariableName=ScopeData4
  Out1 : Outport
  wires:
  Saturation/1 -> Add/2
  Add/1 -> Out1/1, Scope/1
  rotational velocity/1 -> Scope1/1, Add/1
  Ramp/1 -> Saturation/1

== system Simulation/Guasti Sensori/Guasto Sensore yaw ==
  rotational velocity : Inport
  Add : Sum
  Ramp : simulink/Sources/Ramp  slope=0.01  start=20  InitialOutput=0
  Saturation : Saturate  UpperLimit=2  LowerLimit=-2
  Scope : Scope
      settings: ActiveDisplayYMinimum=-0.46753979424554504  ActiveDisplayYMaximum=0.86875215367157943  DataLoggingVariableName=ScopeData3
  Scope1 : Scope
      settings: ActiveDisplayYMinimum=-0.55531902367440134  ActiveDisplayYMaximum=0.70340368575655188  DataLoggingVariableName=ScopeData4
  Out1 : Outport
  wires:
  Add/1 -> Scope/1, Out1/1
  rotational velocity/1 -> Scope1/1, Add/1
  Ramp/1 -> Saturation/1
  Saturation/1 -> Add/2

== system Simulation/Guasti Sensori1/Guasto X ==
  rotational velocity : Inport
  Add : Sum
  Ramp : simulink/Sources/Ramp  slope=0.02  start=20  InitialOutput=0
  Saturation : Saturate  UpperLimit=5  LowerLimit=-5
  Scope : Scope
      settings: ActiveDisplayYMinimum=-0.47156763154329079  ActiveDisplayYMaximum=0.958434860305525  DataLoggingVariableName=ScopeData3
  Scope1 : Scope
      settings: ActiveDisplayYMinimum=-12.060004965377948  ActiveDisplayYMaximum=2.3420345775206344  DataLoggingVariableName=ScopeData4
  Out1 : Outport
  wires:
  Add/1 -> Out1/1, Scope/1
  rotational velocity/1 -> Add/1, Scope1/1
  Ramp/1 -> Saturation/1
  Saturation/1 -> Add/2

== system Simulation/Guasti Sensori1/Guasto Y ==
  In1 : Inport
  Add : Sum
  Ramp : simulink/Sources/Ramp  slope=0.02  start=20  InitialOutput=0
  Saturation : Saturate  UpperLimit=5  LowerLimit=-5
  Scope : Scope
      settings: ActiveDisplayYMinimum=-1  ActiveDisplayYMaximum=1  DataLoggingVariableName=ScopeData3
  Scope1 : Scope
      settings: ActiveDisplayYMinimum=-0.55531902367440134  ActiveDisplayYMaximum=0.70340368575655188  DataLoggingVariableName=ScopeData4
  Out1 : Outport
  wires:
  Add/1 -> Scope/1, Out1/1
  In1/1 -> Scope1/1, Add/1
  Ramp/1 -> Saturation/1
  Saturation/1 -> Add/2

== system Simulation/Guasti Sensori1/Guasto Z ==
  rotational velocity : Inport
  Add : Sum
  Ramp : simulink/Sources/Ramp  slope=0.02  start=20  InitialOutput=0
  Saturation : Saturate  UpperLimit=2  LowerLimit=-2
  Scope : Scope
      settings: ActiveDisplayYMinimum=-0.46753979424554504  ActiveDisplayYMaximum=0.86875215367157943  DataLoggingVariableName=ScopeData3
  Scope1 : Scope
      settings: ActiveDisplayYMinimum=-0.55531902367440134  ActiveDisplayYMaximum=0.70340368575655188  DataLoggingVariableName=ScopeData4
  Out1 : Outport
  wires:
  Add/1 -> Scope/1, Out1/1
  rotational velocity/1 -> Scope1/1, Add/1
  Ramp/1 -> Saturation/1
  Saturation/1 -> Add/2

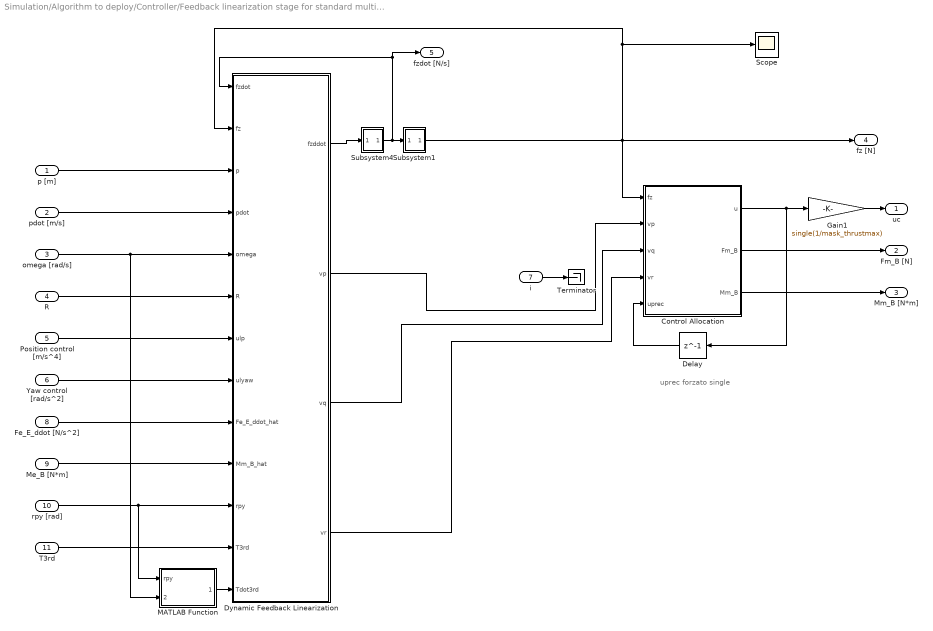
== system Simulation/Algorithm to deploy/Controller/Feedback linearization stage for standard multirotors ==
  note: uprec forzato single
  p [m] : Inport
  pdot [m/s] : Inport  Port=2
  omega [rad/s] : Inport  Port=3
  R : Inport  Port=4
  Position control [m/s^4] : Inport  Port=5
  Yaw control [rad/s^2] : Inport  Port=6
  i : Inport  Port=7
  Fe_E_ddot [N/s^2] : Inport  Port=8
  Me_B [N*m] : Inport  Port=9
  rpy [rad] : Inport  Port=10
  T3rd : Inport  Port=11
  Control Allocation : MATLAB Function  TreatAsAtomicUnit=on
  Delay : Delay  DelayLength=1  InitialCondition=0
  Dynamic Feedback Linearization : MATLAB Function  TreatAsAtomicUnit=on
  Gain1 : Gain  Gain=single(1/mask_thrustmax)
  MATLAB Function : MATLAB Function  TreatAsAtomicUnit=on
  Scope : Scope
      settings: ActiveDisplayYMinimum=13.64532  ActiveDisplayYMaximum=29.09214
  Subsystem1 : Subsystem  mask{mask_IC=single(mask_m*mask_g), mask_ts=mask_Ts}
      mask prompts: mask_IC "Initial condition"; mask_ts "Sample time"
      mask DialogControl DescGroupVar Prompt: Backward Euler integrator
      mask DialogControl DescTextVar Prompt: Discrete time block approximating an integrator through backward Euler.
  Subsystem4 : Subsystem  mask{mask_IC=single(zeros(1,1)), mask_ts=mask_Ts}
      mask prompts: mask_IC "Initial condition"; mask_ts "Sample time"
      mask DialogControl DescGroupVar Prompt: Backward Euler integrator
      mask DialogControl DescTextVar Prompt: Discrete time block approximating an integrator through backward Euler.
  Terminator : Terminator
  uc : Outport  PortDimensions=mask_na
  Fm_B [N] : Outport  Port=2  PortDimensions=3
  Mm_B [N*m] : Outport  Port=3  PortDimensions=3
  fz [N] : Outport  Port=4
  fzdot [N/s] : Outport  Port=5
  wires:
  omega [rad/s]/1 -> MATLAB Function/2(omega), Dynamic Feedback Linearization/5(omega)
  pdot [m/s]/1 -> Dynamic Feedback Linearization/4(pdot)
  R/1 -> Dynamic Feedback Linearization/6(R)
  p [m]/1 -> Dynamic Feedback Linearization/3(p)
  Dynamic Feedback Linearization/1(fzddot) -> Subsystem4/1(In1)
  Subsystem4/1(Out1) -> Subsystem1/1(In1), fzdot [N/s]/1, Dynamic Feedback Linearization/1(fzdot)
  Dynamic Feedback Linearization/3(vq) -> Control Allocation/3(vq)
  Subsystem1/1(Out1) -> Dynamic Feedback Linearization/2(fz), Scope/1, fz [N]/1, Control Allocation/1(fz)
  Dynamic Feedback Linearization/2(vp) -> Control Allocation/2(vp)
  Dynamic Feedback Linearization/4(vr) -> Control Allocation/4(vr)
  Delay/1 -> Control Allocation/5(uprec)
  Control Allocation/3(Mm_B) -> Mm_B [N*m]/1
  Control Allocation/1(u) -> Gain1/1, Delay/1
  Control Allocation/2(Fm_B) -> Fm_B [N]/1
  Gain1/1 -> uc/1
  Position control [m/s^4]/1 -> Dynamic Feedback Linearization/7(ulp)
  Yaw control [rad/s^2]/1 -> Dynamic Feedback Linearization/8(ulyaw)
  Me_B [N*m]/1 -> Dynamic Feedback Linearization/10(Mm_B_hat)
  Fe_E_ddot [N/s^2]/1 -> Dynamic Feedback Linearization/9(Fe_E_ddot_hat)
  i/1 -> Terminator/1
  rpy [rad]/1 -> Dynamic Feedback Linearization/11(rpy), MATLAB Function/1(rpy)
  T3rd/1 -> Dynamic Feedback Linearization/12(T3rd)
  MATLAB Function/1(Tdot3rd) -> Dynamic Feedback Linearization/13(Tdot3rd)

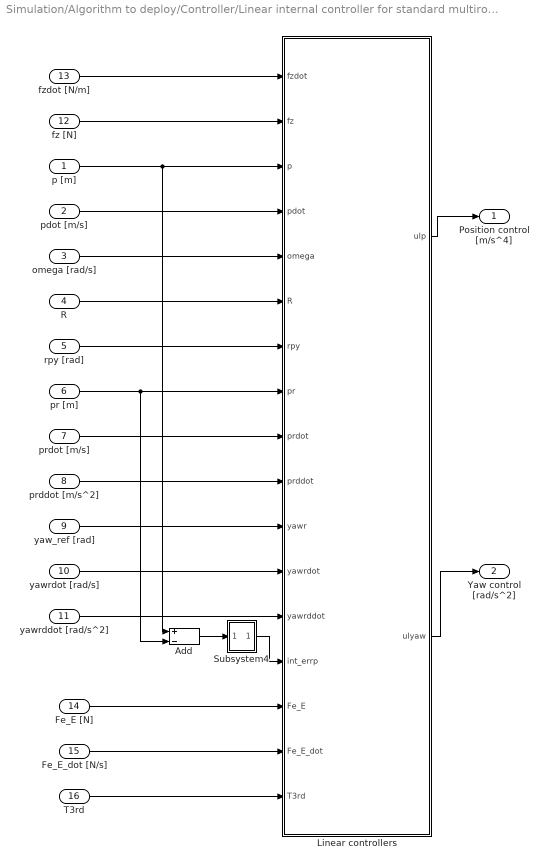
== system Simulation/Algorithm to deploy/Controller/Linear internal controller for standard multirotors ==
  p [m] : Inport
  pdot [m/s] : Inport  Port=2
  omega [rad/s] : Inport  Port=3
  R : Inport  Port=4
  rpy [rad] : Inport  Port=5
  pr [m] : Inport  Port=6
  prdot [m/s] : Inport  Port=7
  prddot [m/s^2] : Inport  Port=8
  yaw_ref [rad] : Inport  Port=9
  yawrdot [rad/s] : Inport  Port=10
  yawrddot [rad/s^2] : Inport  Port=11
  fz [N] : Inport  Port=12
  fzdot [N/m] : Inport  Port=13
  Fe_E [N] : Inport  Port=14
  Fe_E_dot [N/s] : Inport  Port=15
  T3rd : Inport  Port=16
  Add : Sum  Inputs=+-
  Linear controllers : MATLAB Function  TreatAsAtomicUnit=on
  Subsystem4 : Subsystem  mask{mask_IC=single(zeros(1,1)), mask_ts=mask_Ts}
      mask prompts: mask_IC "Initial condition"; mask_ts "Sample time"
      mask DialogControl DescGroupVar Prompt: Backward Euler integrator
      mask DialogControl DescTextVar Prompt: Discrete time block approximating an integrator through backward Euler.
  " Position control [m/s^4]" : Outport
  " Yaw control [rad/s^2]" : Outport  Port=2
  wires:
  omega [rad/s]/1 -> Linear controllers/5(omega)
  pr [m]/1 -> Add/2, Linear controllers/8(pr)
  pdot [m/s]/1 -> Linear controllers/4(pdot)
  R/1 -> Linear controllers/6(R)
  p [m]/1 -> Add/1, Linear controllers/3(p)
  prddot [m/s^2]/1 -> Linear controllers/10(prddot)
  prdot [m/s]/1 -> Linear controllers/9(prdot)
  yaw_ref [rad]/1 -> Linear controllers/11(yawr)
  yawrdot [rad/s]/1 -> Linear controllers/12(yawrdot)
  yawrddot [rad/s^2]/1 -> Linear controllers/13(yawrddot)
  Add/1 -> Subsystem4/1(In1)
  Subsystem4/1(Out1) -> Linear controllers/14(int_errp)
  Linear controllers/1(ulp) -> " Position control [m/s^4]"/1
  Linear controllers/2(ulyaw) -> " Yaw control [rad/s^2]"/1
  fzdot [N/m]/1 -> Linear controllers/1(fzdot)
  fz [N]/1 -> Linear controllers/2(fz)
  rpy [rad]/1 -> Linear controllers/7(rpy)
  Fe_E_dot [N/s]/1 -> Linear controllers/16(Fe_E_dot)
  Fe_E [N]/1 -> Linear controllers/15(Fe_E)
  T3rd/1 -> Linear controllers/17(T3rd)

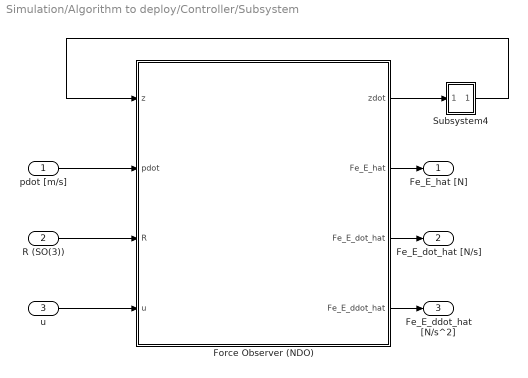
== system Simulation/Algorithm to deploy/Controller/Subsystem ==
  pdot [m/s] : Inport
  R (SO(3)) : Inport  Port=2
  u : Inport  Port=3
  Force Observer (NDO) : MATLAB Function  TreatAsAtomicUnit=on
  Subsystem4 : Subsystem  mask{mask_IC=single(zeros(mask_nzeta,1)), mask_ts=mask_Ts}
      mask prompts: mask_IC "Initial condition"; mask_ts "Sample time"
      mask DialogControl DescGroupVar Prompt: Backward Euler integrator
      mask DialogControl DescTextVar Prompt: Discrete time block approximating an integrator through backward Euler.
  Fe_E_hat [N] : Outport
  Fe_E_dot_hat [N/s] : Outport  Port=2
  Fe_E_ddot_hat [N/s^2] : Outport  Port=3
  wires:
  Force Observer (NDO)/1(zdot) -> Subsystem4/1(In1)
  Force Observer (NDO)/3(Fe_E_dot_hat) -> Fe_E_dot_hat [N/s]/1
  Subsystem4/1(Out1) -> Force Observer (NDO)/1(z)
  Force Observer (NDO)/2(Fe_E_hat) -> Fe_E_hat [N]/1
  u/1 -> Force Observer (NDO)/4(u)
  Force Observer (NDO)/4(Fe_E_ddot_hat) -> Fe_E_ddot_hat [N/s^2]/1
  pdot [m/s]/1 -> Force Observer (NDO)/2(pdot)
  R (SO(3))/1 -> Force Observer (NDO)/3(R)

== system Simulation/Algorithm to deploy/Controller/Subsystem1 ==
  omega [rad/s] : Inport
  u : Inport  Port=2
  Force Observer (NDO) : MATLAB Function  TreatAsAtomicUnit=on
  Subsystem4 : Subsystem  mask{mask_IC=single(zeros(mask_nzeta,1)), mask_ts=mask_Ts}
      mask prompts: mask_IC "Initial condition"; mask_ts "Sample time"
      mask DialogControl DescGroupVar Prompt: Backward Euler integrator
      mask DialogControl DescTextVar Prompt: Discrete time block approximating an integrator through backward Euler.
  Me_B_hat [N*m] : Outport
  Me_B_dot_hat [N*m/s] : Outport  Port=2
  Me_B_ddot_hat [N*m/s^2] : Outport  Port=3
  wires:
  omega [rad/s]/1 -> Force Observer (NDO)/2(omega)
  Force Observer (NDO)/4(Me_B_ddot_hat) -> Me_B_ddot_hat [N*m/s^2]/1
  u/1 -> Force Observer (NDO)/3(u)
  Force Observer (NDO)/2(Me_B_hat) -> Me_B_hat [N*m]/1
  Subsystem4/1(Out1) -> Force Observer (NDO)/1(z)
  Force Observer (NDO)/3(Me_B_dot_hat) -> Me_B_dot_hat [N*m/s]/1
  Force Observer (NDO)/1(zdot) -> Subsystem4/1(In1)

== system Simulation/Algorithm to deploy/Controller/Feedback linearization stage for standard multirotors/Subsystem1 ==
  In1 : Inport
  Add : Sum  OutDataTypeStr=single
  Delay : Delay  DelayLength=1  InitialCondition=mask_IC
  Delay1 : Delay  DelayLength=1  InitialCondition=0*mask_IC
  Gain : Gain  Gain=single(mask_ts)
  Out1 : Outport
  wires:
  Delay/1 -> Add/1
  Delay1/1 -> Add/2
  In1/1 -> Gain/1
  Gain/1 -> Delay1/1
  Add/1 -> Delay/1, Out1/1

== system Simulation/Algorithm to deploy/Controller/Feedback linearization stage for standard multirotors/Subsystem4 ==
  In1 : Inport
  Add : Sum  OutDataTypeStr=single
  Delay : Delay  DelayLength=1  InitialCondition=mask_IC
  Delay1 : Delay  DelayLength=1  InitialCondition=0*mask_IC
  Gain : Gain  Gain=single(mask_ts)
  Out1 : Outport
  wires:
  Add/1 -> Out1/1, Delay/1
  Gain/1 -> Delay1/1
  In1/1 -> Gain/1
  Delay1/1 -> Add/2
  Delay/1 -> Add/1

== system Simulation/Algorithm to deploy/Controller/Linear internal controller for standard multirotors/Subsystem4 ==
  In1 : Inport
  Add : Sum  OutDataTypeStr=single
  Delay : Delay  DelayLength=1  InitialCondition=mask_IC
  Delay1 : Delay  DelayLength=1  InitialCondition=0*mask_IC
  Gain : Gain  Gain=single(mask_ts)
  Out1 : Outport
  wires:
  Add/1 -> Out1/1, Delay/1
  Gain/1 -> Delay1/1
  In1/1 -> Gain/1
  Delay1/1 -> Add/2
  Delay/1 -> Add/1

== system Simulation/Algorithm to deploy/Controller/Subsystem/Subsystem4 ==
  In1 : Inport
  Add : Sum  OutDataTypeStr=single
  Delay : Delay  DelayLength=1  InitialCondition=mask_IC
  Delay1 : Delay  DelayLength=1  InitialCondition=0*mask_IC
  Gain : Gain  Gain=single(mask_ts)
  Out1 : Outport
  wires:
  Add/1 -> Out1/1, Delay/1
  Gain/1 -> Delay1/1
  In1/1 -> Gain/1
  Delay1/1 -> Add/2
  Delay/1 -> Add/1

== system Simulation/Algorithm to deploy/Controller/Subsystem1/Subsystem4 ==
  In1 : Inport
  Add : Sum  OutDataTypeStr=single
  Delay : Delay  DelayLength=1  InitialCondition=mask_IC
  Delay1 : Delay  DelayLength=1  InitialCondition=0*mask_IC
  Gain : Gain  Gain=single(mask_ts)
  Out1 : Outport
  wires:
  Delay/1 -> Add/1
  Delay1/1 -> Add/2
  In1/1 -> Gain/1
  Gain/1 -> Delay1/1
  Add/1 -> Delay/1, Out1/1

== matlab function Simulation/Fault Detection (FD) Module/Evaluator/MATLAB Function4 ==
  settings: updateMethod=DISCRETE  sampleTime=0.01
  data: raw_alarm input; confirmed_alarm output
function confirmed_alarm = debounce_logic(raw_alarm)
%#codegen
% DEBOUNCE CORTO PER FILTRO LEAD:
% Cattura il picco istantaneo e conferma l'allarme se il picco persiste 
% per almeno 0.1 secondi.

    % Parametri del debounce
    sample_time = 0.001; % Tempo di campionamento (modifica se usi Ts diverso)
    window_size = 0.1;   % FINESTRA CORTA: 0.1 secondi!

    % Timer persistente in memoria
    persistent timer
    if isempty(timer)
        timer = 0;
    end

    confirmed_alarm = 0;

    % Logica del cronometro cumulativo
    if raw_alarm == 1
        timer = timer + sample_time; % Il picco è sopra la soglia
    else
        timer = 0; % Sotto la soglia, azzera il timer
    end

    % Scatto dell'allarme confermato (Sezione Latch/Memoria)
    % Usiamo un persistent latch per far sì che, una volta scattato l'allarme,
    % rimanga acceso anche se il picco del filtro Lead scompare.
    persistent latch_alarm
    if isempty(latch_alarm)
        latch_alarm = 0;
    end

    if timer >= window_size
        latch_alarm = 1; % GUASTO CONFERMATO E MEMORIZZATO
    end

    confirmed_alarm = latch_alarm;
end

== matlab function Simulation/Algorithm to deploy/Controller/Feedback linearization stage for standard multirotors/Control Allocation ==
  data: fz input; vp input; vq input; vr input; u output; uprec input single; mask_J parameter; A_pinv parameter; Fm_B output; Mm_B output; mask_na parameter
function [u,Fm_B,Mm_B] = ControlAllocation(fz,vp,vq,vr,uprec, mask_J,A_pinv,mask_na)

Fm_B = [0; 0; -fz];
Mm_B = mask_J*[vp; vq; vr];
b = [-fz; Mm_B];

% Calculation of forces
u = A_pinv*b;

end

== matlab function Simulation/Fault Detection (FD) Module/Evaluator/MATLAB Function1 ==
  settings: updateMethod=DISCRETE  sampleTime=0.01
  data: raw_alarm input; confirmed_alarm output; current_time input; T_debounce parameter
function confirmed_alarm = debounce_logic(raw_alarm, current_time, T_debounce)
    % DEBOUNCE_LOGIC: Valida un allarme solo se rimane attivo per T_debounce secondi.
    
    % Definiamo le variabili "persistent". 
    % In Simulink, una variabile persistent ricorda il suo valore al ciclo 
    % di calcolo successivo (si comporta come la memoria di un flip-flop).
    persistent timer_start
    persistent is_timing
    
    % Inizializzazione: al tempo t=0, le variabili sono vuote
    if isempty(timer_start)
        timer_start = 0;       % Memoria del tempo in cui l'allarme è scattato
        is_timing = false;     % Flag: il cronometro sta girando?
    end
    
    % Di default, l'allarme confermato è sempre spento (0)
    confirmed_alarm = 0;
    
    % LOGICA DI VALUTAZIONE
    if raw_alarm == 1
        % L'errore grezzo ha superato la soglia!
        
        if ~is_timing
            % Se il cronometro era fermo, lo facciamo partire ORA
            timer_start = current_time;
            is_timing = true;
        end
        
        % Controlliamo da quanto tempo sta suonando l'allarme grezzo
        tempo_trascorso = current_time - timer_start;
        
        if tempo_trascorso >= T_debounce
            % Il tempo è scaduto! L'allarme è reale e confermato.
            confirmed_alarm = 1;
        end
        
    else
        % L'errore grezzo è tornato a 0 (sotto la soglia).
        % Potrebbe essere stato un falso allarme o il guasto è rientrato.
        % RESETTIAMO IL CRONOMETRO.
        is_timing = false;
        confirmed_alarm = 0;
    end
end
